simulink model "chap10_2sim"  (Simulink 5.1)
settings: Solver=ode4  SolverMode=SingleTasking  StartTime=0.0  StopTime=6  FixedStep=0.001  RelTol=1e-3
libraries: simulink x1
settings Model: LastModifiedBy=liu  ExtModeTrigMode=oneshot  ExtModeArmWhenConnect=off  LimitDataPoints=off  ProdHWDeviceType=Microprocessor

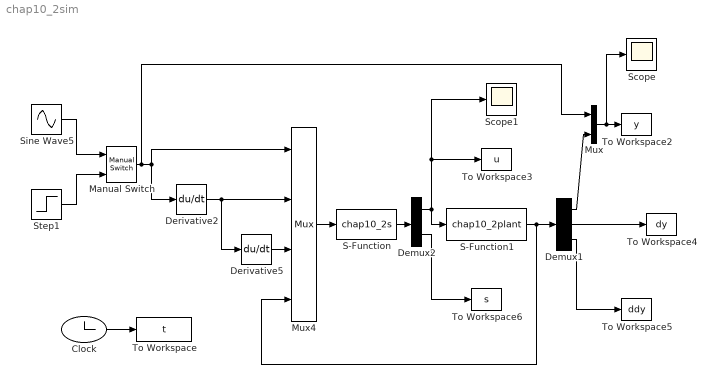
== system chap10_2sim ==
  Clock : Clock
  Demux1 : Demux  Outputs=3
  Demux2 : Demux  Outputs=2
  Derivative2 : Derivative
  Derivative5 : Derivative
  Manual Switch : simulink/Signal Routing/Manual Switch  sw=1  action=0
  Mux : Mux  Inputs=2
  Mux4 : Mux
  S-Function : S-Function  FunctionName=chap10_2s
  S-Function1 : S-Function  FunctionName=chap10_2plant
  Scope : Scope
      settings: YMin=-0.5  YMax=0.5
  Scope1 : Scope
      settings: YMin=-125  YMax=125
  Sine Wave5 : Sin  Amplitude=0.50  Frequency=1*2*pi  SampleTime=0
  Step1 : Step  Time=0  SampleTime=0
  To Workspace : ToWorkspace  VariableName=t  SampleTime=-1  SaveFormat=Array
  To Workspace2 : ToWorkspace  VariableName=y  SampleTime=-1  SaveFormat=Array
  To Workspace3 : ToWorkspace  VariableName=u  SampleTime=-1  SaveFormat=Array
  To Workspace4 : ToWorkspace  VariableName=dy  SampleTime=-1  SaveFormat=Array
  To Workspace5 : ToWorkspace  VariableName=ddy  SampleTime=-1  SaveFormat=Array
  To Workspace6 : ToWorkspace  VariableName=s  SampleTime=-1  SaveFormat=Array
  wires:
  Sine Wave5/1 -> Manual Switch/1
  Step1/1 -> Manual Switch/2
  Mux4/1 -> S-Function/1
  Derivative5/1 -> Mux4/3
  Derivative2/1 -> Mux4/2, Derivative5/1
  Manual Switch/1 -> Mux4/1, Derivative2/1, Mux/1
  S-Function/1 -> Demux2/1
  Clock/1 -> To Workspace/1
  Demux2/1 -> S-Function1/1, To Workspace3/1, Scope1/1
  Demux2/2 -> To Workspace6/1
  Mux/1 -> To Workspace2/1, Scope/1
  Demux1/1 -> Mux/2
  Demux1/3 -> To Workspace5/1
  Demux1/2 -> To Workspace4/1
  S-Function1/1 -> Demux1/1, Mux4/4
